simulink model "Comp_FDC_main"  (R2021b)
settings: Solver=FixedStepDiscrete  StartTime=0.0  StopTime=10.0  RelTol=1e-3  EnableMultiTasking=on
settings Model: DataDictionary=APPTypes.sldd  Creator=FVT22063  LastModifiedBy=FVT22063
settings SolverCC: AutoInsertRateTranBlk=on
settings DataIOCC: SaveFormat=StructureWithTime
settings OptimizationCC: DefaultParameterBehavior=Inlined  EnhancedBackFolding=on  PassReuseOutputArgsAs=Individual arguments  ZeroExternalMemoryAtStartup=off  ZeroInternalMemoryAtStartup=off  OptimizeBlockOrder=speed  DifferentSizesBufferReuse=on  OptimizationCustomize=off  EfficientTunableParamExpr=on
settings DebuggingCC: ParameterTunabilityLossMsg=error
settings ModelReferenceCC: ModelReferenceNumInstancesAllowed=Single
settings SFSimCC: MATLABDynamicMemAlloc=off
settings RTWCC: Description=AUTOSAR  SystemTargetFile=autosar.tlc  GenCodeOnly=on  TemplateMakefile=ert_default_tmf
settings CodeAppCC: ForceParamTrailComments=on  IgnoreCustomStorageClasses=off  OperatorAnnotations=on  SimulinkDataObjDesc=on  SFDataObjDesc=on  InsertBlockDesc=on
settings STFCustomTargetCC: TargetLangStandard=C99 (ISO)  MultiwordLength=256  ParMdlRefBuildCompliant=on  CompOptLevelCompliant=on  IncludeMdlTerminateFcn=off  CombineOutputUpdateFcns=on  SuppressErrorStatus=on  ERTCustomFileBanners=on  SupportNonFinite=off  SupportComplex=off  SupportContinuousTime=off  SupportNonInlinedSFcns=off  RemoveResetFunc=on  MATLABClassNameForMDSCustomization=Simulink.SoftwareTarget.ERTCustomization  AutosarCompliant=on  GRTInterface=off  UseToolchainInfoCompliant=on  LookupTableObjectStructAxisOrder=2,1,3,4,...  LUTObjectStructOrderEvenSpacing=Size,Table,Breakpoints  SystemTargetFile=autosar.tlc
settings ERTTargetCC: TargetLangStandard=C99 (ISO)  ConcurrentExecutionCompliant=off  IncludeMdlTerminateFcn=off  SuppressErrorStatus=on  SupportNonFinite=off  SupportComplex=off  ModelStepFunctionPrototypeControlCompliant=off  CPPClassGenCompliant=off  AutosarCompliant=on  LookupTableObjectStructAxisOrder=2,1,3,4,...  LUTObjectStructOrderEvenSpacing=Size,Table,Breakpoints  InlinedParameterPlacement=NonHierarchical  ERTCustomFileTemplate=example_file_process.tlc

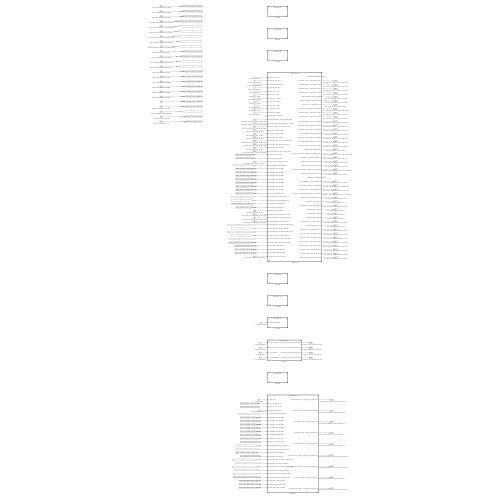
[thumbnail: Simulink's stored preview of the top-level diagram]
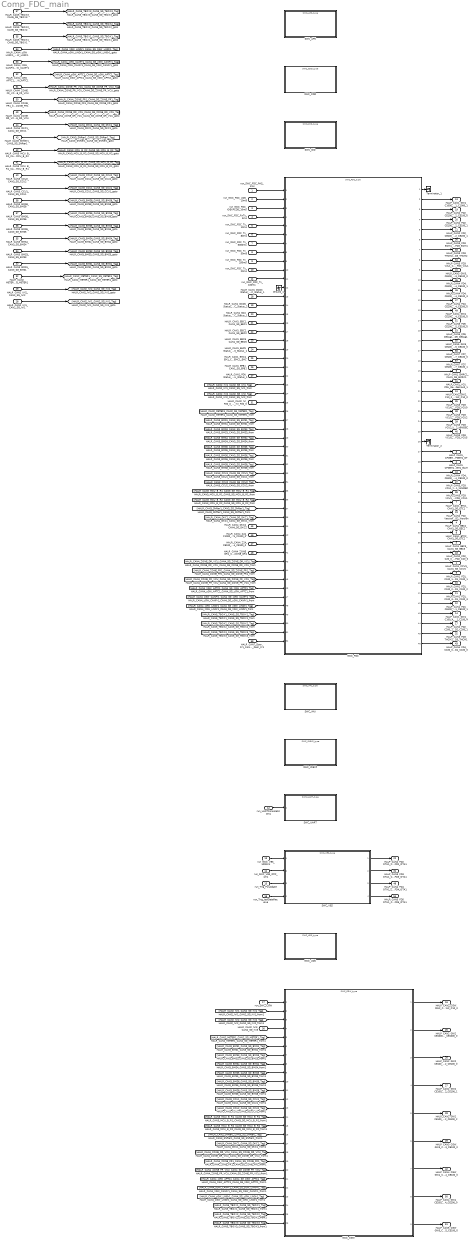
== system Comp_FDC_main ==
  run_SWC_FDC_PAS_1ms : Inport  SampleTime=0.001  OutputFunctionCall=on
  run_SWC_FDC_UDS_10ms : Inport  Port=2  SampleTime=0.01  OutputFunctionCall=on
  run_SWC_FDC_IOEXPCDD_10ms : Inport  Port=3  SampleTime=0.01  OutputFunctionCall=on
  run_SWC_FDC_RxTx_5ms : Inport  Port=4  SampleTime=0.005  OutputFunctionCall=on
  run_SWC_FDC_Tx_10ms : Inport  Port=5  SampleTime=0.01  OutputFunctionCall=on
  run_SWC_FDC_Tx_80ms : Inport  Port=6  SampleTime=0.08  OutputFunctionCall=on
  run_SWC_FDC_Tx_5000ms : Inport  Port=7  SampleTime=5  OutputFunctionCall=on
  run_SWC_FDC_Tx_50ms : Inport  Port=8  SampleTime=0.05  OutputFunctionCall=on
  run_SWC_FDC_Tx_250ms : Inport  Port=9  SampleTime=0.25  OutputFunctionCall=on
  run_SWC_FDC_Tx_20ms : Inport  Port=10  SampleTime=0.02  OutputFunctionCall=on
  run_SWC_FDC_Tx_100ms : Inport  Port=11  SampleTime=0.1  OutputFunctionCall=on
  run_UARTConsole100ms : Inport  Port=12  SampleTime=0.1  OutputFunctionCall=on
  run_SWC_VES_1000ms : Inport  Port=13  SampleTime=1  OutputFunctionCall=on
  run_SWC_VES_IPCF_1ms : Inport  Port=14  SampleTime=0.001  OutputFunctionCall=on
  run_Trig_FwUpdate : Inport  Port=15  OutputFunctionCall=on
  run_Trig_IpcfDataReceive : Inport  Port=16  OutputFunctionCall=on
  run_SWC_CGW : Inport  Port=17  OutputFunctionCall=on
  HALR_CAN1_DCDC_Status_1_CAN1_SG_DCDC_Status_1 : Inport  Port=18  OutDataTypeStr=Bus: DT_CAN1_SG_DCDC_Status_1  PortDimensions=1  BusOutputAsStruct=on
  HALR_CAN1_DCDC_Status_2_CAN1_SG_DCDC_Status_2 : Inport  Port=19  OutDataTypeStr=Bus: DT_CAN1_SG_DCDC_Status_2  PortDimensions=1  BusOutputAsStruct=on
  HALR_CAN1_EAC_Status_1_CAN1_SG_EAC_Status_1 : Inport  Port=20  OutDataTypeStr=Bus: DT_CAN1_SG_EAC_Status_1  PortDimensions=1  BusOutputAsStruct=on
  HALR_CAN1_EBC1_CAN1_SG_EBC1 : Inport  Port=21  OutDataTypeStr=Bus: DT_CAN1_SG_EBC1  PortDimensions=1  BusOutputAsStruct=on
  HALR_CAN1_EBC2_CAN1_SG_EBC2 : Inport  Port=22  OutDataTypeStr=Bus: DT_CAN1_SG_EBC2  PortDimensions=1  BusOutputAsStruct=on
  HALR_CAN1_EBC5_CAN1_SG_EBC5 : Inport  Port=23  OutDataTypeStr=Bus: DT_CAN1_SG_EBC5  PortDimensions=1  BusOutputAsStruct=on
  HALR_CAN1_EHPS_Status_1_CAN1_SG_EHPS_Status_1 : Inport  Port=24  OutDataTypeStr=Bus: DT_CAN1_SG_EHPS_Status_1  PortDimensions=1  BusOutputAsStruct=on
  HALR_CAN1_EMC1_EM1_CAN1_SG_EMC1_EM1 : Inport  Port=25  OutDataTypeStr=Bus: DT_CAN1_SG_EMC1_EM1  PortDimensions=1  BusOutputAsStruct=on
  HALR_CAN1_EPB1_CAN1_SG_EPB1 : Inport  Port=26  OutDataTypeStr=Bus: DT_CAN1_SG_EPB1  PortDimensions=1  BusOutputAsStruct=on
  HALR_CAN1_PDU_Status_1_CAN1_SG_PDU_Status_1 : Inport  Port=27  OutDataTypeStr=Bus: DT_CAN1_SG_PDU_Status_1  PortDimensions=1  BusOutputAsStruct=on
  HALR_CAN2_IVI1_CAN2_SG_IVI1 : Inport  Port=28  OutDataTypeStr=Bus: DT_CAN2_SG_IVI1  PortDimensions=1  BusOutputAsStruct=on
  HALR_CAN2_IVI2_CAN2_SG_IVI2 : Inport  Port=29  OutDataTypeStr=Bus: DT_CAN2_SG_IVI2  PortDimensions=1  BusOutputAsStruct=on
  HALR_CAN2_IVI3_CAN2_SG_IVI3 : Inport  Port=30  OutDataTypeStr=Bus: DT_CAN2_SG_IVI3  PortDimensions=1  BusOutputAsStruct=on
  HALR_CAN2_IVI_P20_0_CAN2_SG_IVI_P20_0 : Inport  Port=31  OutDataTypeStr=Bus: DT_CAN2_SG_IVI_P20_0  PortDimensions=1  BusOutputAsStruct=on
  HALR_CAN2_METER1_CAN2_SG_METER1 : Inport  Port=32  OutDataTypeStr=Bus: DT_CAN2_SG_METER1  PortDimensions=1  BusOutputAsStruct=on
  HALR_CAN3_BMS1_CAN3_SG_BMS1 : Inport  Port=33  OutDataTypeStr=Bus: DT_CAN3_SG_BMS1  PortDimensions=1  BusOutputAsStruct=on
  HALR_CAN3_BMS3_CAN3_SG_BMS3 : Inport  Port=34  OutDataTypeStr=Bus: DT_CAN3_SG_BMS3  PortDimensions=1  BusOutputAsStruct=on
  HALR_CAN3_BMS4_CAN3_SG_BMS4 : Inport  Port=35  OutDataTypeStr=Bus: DT_CAN3_SG_BMS4  PortDimensions=1  BusOutputAsStruct=on
  HALR_CAN3_BMS5_CAN3_SG_BMS5 : Inport  Port=36  OutDataTypeStr=Bus: DT_CAN3_SG_BMS5  PortDimensions=1  BusOutputAsStruct=on
  HALR_CAN3_BMS6_CAN3_SG_BMS6 : Inport  Port=37  OutDataTypeStr=Bus: DT_CAN3_SG_BMS6  PortDimensions=1  BusOutputAsStruct=on
  HALR_CAN3_BMS8_CAN3_SG_BMS8 : Inport  Port=38  OutDataTypeStr=Bus: DT_CAN3_SG_BMS8  PortDimensions=1  BusOutputAsStruct=on
  HALR_CAN3_CCU1_CAN3_SG_CCU1 : Inport  Port=39  OutDataTypeStr=Bus: DT_CAN3_SG_CCU1  PortDimensions=1  BusOutputAsStruct=on
  HALR_CAN3_CCU2_CAN3_SG_CCU2 : Inport  Port=40  OutDataTypeStr=Bus: DT_CAN3_SG_CCU2  PortDimensions=1  BusOutputAsStruct=on
  HALR_CAN3_MCU_B_R1_CAN3_SG_MCU_B_R1 : Inport  Port=41  OutDataTypeStr=Bus: DT_CAN3_SG_MCU_B_R1  PortDimensions=1  BusOutputAsStruct=on
  HALR_CAN3_MCU_B_R2_CAN3_SG_MCU_B_R2 : Inport  Port=42  OutDataTypeStr=Bus: DT_CAN3_SG_MCU_B_R2  PortDimensions=1  BusOutputAsStruct=on
  HALR_CAN3_Shifter1_CAN3_SG_Shifter1 : Inport  Port=43  OutDataTypeStr=Bus: DT_CAN3_SG_Shifter1  PortDimensions=1  BusOutputAsStruct=on
  HALR_CAN4_DKC1_CAN4_SG_DKC1 : Inport  Port=44  OutDataTypeStr=Bus: DT_CAN4_SG_DKC1  PortDimensions=1  BusOutputAsStruct=on
  HALR_CAN4_DKC2_CAN4_SG_DKC2 : Inport  Port=45  OutDataTypeStr=Bus: DT_CAN4_SG_DKC2  PortDimensions=1  BusOutputAsStruct=on
  HALR_CAN4_Z24_C1000_0_CAN4_SG_Z24_C1000_0 : Inport  Port=46  OutDataTypeStr=Bus: DT_CAN4_SG_Z24_C1000_0  PortDimensions=1  BusOutputAsStruct=on
  HALR_CAN4_Z24_CE100_0_CAN4_SG_Z24_CE100_0 : Inport  Port=47  OutDataTypeStr=Bus: DT_CAN4_SG_Z24_CE100_0  PortDimensions=1  BusOutputAsStruct=on
  HALR_CAN4_ZONE_DR1_CAN4_SG_ZONE_DR1 : Inport  Port=48  OutDataTypeStr=Bus: DT_CAN4_SG_ZONE_DR1  PortDimensions=1  BusOutputAsStruct=on
  HALR_CAN4_ZONE_DR_VCU_CAN4_SG_ZONE_DR_VCU : Inport  Port=49  OutDataTypeStr=Bus: DT_CAN4_SG_ZONE_DR_VCU  PortDimensions=1  BusOutputAsStruct=on
  HALR_CAN4_ZONE_FR1_CAN4_SG_ZONE_FR1 : Inport  Port=50  OutDataTypeStr=Bus: DT_CAN4_SG_ZONE_FR1  PortDimensions=1  BusOutputAsStruct=on
  HALR_CAN4_ZONE_FR_VCU_CAN4_SG_ZONE_FR_VCU : Inport  Port=51  OutDataTypeStr=Bus: DT_CAN4_SG_ZONE_FR_VCU  PortDimensions=1  BusOutputAsStruct=on
  HALR_CAN4_zGW_APTC1_CAN4_SG_zGW_APTC1 : Inport  Port=52  OutDataTypeStr=Bus: DT_CAN4_SG_zGW_APTC1  PortDimensions=1  BusOutputAsStruct=on
  HALR_CAN4_zGW_CANFr1_CAN4_SG_zGW_CANFr1 : Inport  Port=53  OutDataTypeStr=Bus: DT_CAN4_SG_zGW_CANFr1  PortDimensions=1  BusOutputAsStruct=on
  HALR_CAN4_zGW_LINDr1_CAN4_SG_zGW_LINDr1 : Inport  Port=54  OutDataTypeStr=Bus: DT_CAN4_SG_zGW_LINDr1  PortDimensions=1  BusOutputAsStruct=on
  HALR_CAN5_TBOX1_CAN5_SG_TBOX1 : Inport  Port=55  OutDataTypeStr=Bus: DT_CAN5_SG_TBOX1  PortDimensions=1  BusOutputAsStruct=on
  HALR_CAN5_TBOX2_CAN5_SG_TBOX2 : Inport  Port=56  OutDataTypeStr=Bus: DT_CAN5_SG_TBOX2  PortDimensions=1  BusOutputAsStruct=on
  HALR_CAN5_TBOX3_CAN5_SG_TBOX3 : Inport  Port=57  OutDataTypeStr=Bus: DT_CAN5_SG_TBOX3  PortDimensions=1  BusOutputAsStruct=on
  HALR_CAN7_Door_Fr1_CAN7_SG_Door_Fr1 : Inport  Port=58  OutDataTypeStr=Bus: DT_CAN7_SG_Door_Fr1  PortDimensions=1  BusOutputAsStruct=on
  Ground_1 : Ground
  SWC_APS : ModelReference  ModelNameDialog=SWC_APS_type  SimulationMode=Normal  ScheduleRates=on  ModelReferenceVersion=1.1
  SWC_CDD : ModelReference  ModelNameDialog=SWC_CDD_type  SimulationMode=Normal  ScheduleRates=on  ModelReferenceVersion=1.1
  SWC_CGW : ModelReference  ModelNameDialog=SWC_CGW_type  SimulationMode=Normal  ScheduleRates=on  ModelReferenceVersion=1.1
  SWC_DID : ModelReference  ModelNameDialog=SWC_DID_type  SimulationMode=Normal  ScheduleRates=on  ModelReferenceVersion=1.1
  SWC_FDC : ModelReference  ModelNameDialog=SWC_FDC_type  SimulationMode=Normal  ScheduleRates=on  ModelReferenceVersion=1.1
  SWC_IMU : ModelReference  ModelNameDialog=SWC_IMU_type  SimulationMode=Normal  ScheduleRates=on  ModelReferenceVersion=1.1
  SWC_IOEXP : ModelReference  ModelNameDialog=SWC_IOEXP_type  SimulationMode=Normal  ScheduleRates=on  ModelReferenceVersion=1.1
  SWC_UART : ModelReference  ModelNameDialog=SWC_UART_type  SimulationMode=Normal  ScheduleRates=on  ModelReferenceVersion=1.1
  SWC_UDS : ModelReference  ModelNameDialog=SWC_UDS_type  SimulationMode=Normal  ScheduleRates=on  ModelReferenceVersion=1.1
  SWC_VES : ModelReference  ModelNameDialog=SWC_VES_type  SimulationMode=Normal  ScheduleRates=on  ModelReferenceVersion=1.1
  Terminator_1 : Terminator
  Terminator_2 : Terminator
  HALP_CAN1_CCVS_CAN1_SG_CCVS : Outport  OutDataTypeStr=Bus: DT_CAN1_SG_CCVS  PortDimensions=1  BusOutputAsStruct=on
  HALP_CAN1_CFGEM1_BAM_CAN1_SG_CFGEM1_BAM : Outport  Port=2  OutDataTypeStr=Bus: DT_CAN1_SG_CFGEM1_BAM  PortDimensions=1  BusOutputAsStruct=on
  HALP_CAN1_CFGEM1_DT_CAN1_SG_CFGEM1_DT : Outport  Port=3  OutDataTypeStr=Bus: DT_CAN1_SG_CFGEM1_DT  PortDimensions=1  BusOutputAsStruct=on
  HALP_CAN1_EEC2_CAN1_SG_EEC2 : Outport  Port=4  OutDataTypeStr=Bus: DT_CAN1_SG_EEC2  PortDimensions=1  BusOutputAsStruct=on
  HALP_CAN1_EEC3_CAN1_SG_EEC3 : Outport  Port=5  OutDataTypeStr=Bus: DT_CAN1_SG_EEC3  PortDimensions=1  BusOutputAsStruct=on
  HALP_CAN1_EMRC1_CAN1_SG_EMRC1 : Outport  Port=6  OutDataTypeStr=Bus: DT_CAN1_SG_EMRC1  PortDimensions=1  BusOutputAsStruct=on
  HALP_CAN1_ETC1_CAN1_SG_ETC1 : Outport  Port=7  OutDataTypeStr=Bus: DT_CAN1_SG_ETC1  PortDimensions=1  BusOutputAsStruct=on
  HALP_CAN1_ETC2_CAN1_SG_ETC2 : Outport  Port=8  OutDataTypeStr=Bus: DT_CAN1_SG_ETC2  PortDimensions=1  BusOutputAsStruct=on
  HALP_CAN1_FD1_C100_1_CAN1_SG_FD1_C100_1 : Outport  Port=9  OutDataTypeStr=Bus: DT_CAN1_SG_FD1_C100_1  PortDimensions=1  BusOutputAsStruct=on
  HALP_CAN1_FD1_C100_2_CAN1_SG_FD1_C100_2 : Outport  Port=10  OutDataTypeStr=Bus: DT_CAN1_SG_FD1_C100_2  PortDimensions=1  BusOutputAsStruct=on
  HALP_CAN1_FD1_C100_3_CAN1_SG_FD1_C100_3 : Outport  Port=11  OutDataTypeStr=Bus: DT_CAN1_SG_FD1_C100_3  PortDimensions=1  BusOutputAsStruct=on
  HALP_CAN1_FD1_CE100_1_CAN1_SG_FD1_CE100_1 : Outport  Port=12  OutDataTypeStr=Bus: DT_CAN1_SG_FD1_CE100_1  PortDimensions=1  BusOutputAsStruct=on
  HALP_CAN1_GW1_C1000_1_CAN1_SG_GW1_C1000_1 : Outport  Port=13  OutDataTypeStr=Bus: DT_CAN1_SG_GW1_C1000_1  PortDimensions=1  BusOutputAsStruct=on
  HALP_CAN1_GW1_C100_4_CAN1_SG_GW1_C100_4 : Outport  Port=14  OutDataTypeStr=Bus: DT_CAN1_SG_GW1_C100_4  PortDimensions=1  BusOutputAsStruct=on
  HALP_CAN1_VCU_PDU_Demand_1_CAN1_SG_VCU_PDU_Demand_1 : Outport  Port=15  OutDataTypeStr=Bus: DT_CAN1_SG_VCU_PDU_Demand_1  PortDimensions=1  BusOutputAsStruct=on
  HALP_CAN2_CGW_GW2_C10_0_CAN2_SG_CGW_GW2_C10_0 : Outport  Port=16  OutDataTypeStr=Bus: DT_CAN2_SG_CGW_GW2_C10_0  PortDimensions=1  BusOutputAsStruct=on
  HALP_CAN2_FD2_C200_1_CAN2_SG_FD2_C200_1 : Outport  Port=17  OutDataTypeStr=Bus: DT_CAN2_SG_FD2_C200_1  PortDimensions=1  BusOutputAsStruct=on
  HALP_CAN2_FD2_C20_0_CAN2_SG_FD2_C20_0 : Outport  Port=18  OutDataTypeStr=Bus: DT_CAN2_SG_FD2_C20_0  PortDimensions=1  BusOutputAsStruct=on
  HALP_CAN2_FD2_CE100_0_CAN2_SG_FD2_CE100_0 : Outport  Port=19  OutDataTypeStr=Bus: DT_CAN2_SG_FD2_CE100_0  PortDimensions=1  BusOutputAsStruct=on
  HALP_CAN2_FD2_CE100_1_CAN2_SG_FD2_CE100_1 : Outport  Port=20  OutDataTypeStr=Bus: DT_CAN2_SG_FD2_CE100_1  PortDimensions=1  BusOutputAsStruct=on
  HALP_CAN2_FD2_CE200_1_CAN2_SG_FD2_CE200_1 : Outport  Port=21  OutDataTypeStr=Bus: DT_CAN2_SG_FD2_CE200_1  PortDimensions=1  BusOutputAsStruct=on
  HALP_CAN2_FD2_OTA1_CAN2_SG_FD2_OTA1 : Outport  Port=22  OutDataTypeStr=Bus: DT_CAN2_SG_FD2_OTA1  PortDimensions=1  BusOutputAsStruct=on
  HALP_CAN2_FD2_Version_CAN2_SG_FD2_Version : Outport  Port=23  OutDataTypeStr=Bus: DT_CAN2_SG_FD2_Version  PortDimensions=1  BusOutputAsStruct=on
  HALP_CAN2_GW2_C10_0_CAN2_SG_GW2_C10_0 : Outport  Port=24  OutDataTypeStr=Bus: DT_CAN2_SG_GW2_C10_0  PortDimensions=1  BusOutputAsStruct=on
  HALP_CAN2_GW2_CE1000_0_CAN2_SG_GW2_CE1000_0 : Outport  Port=25  OutDataTypeStr=Bus: DT_CAN2_SG_GW2_CE1000_0  PortDimensions=1  BusOutputAsStruct=on
  HALP_CAN2_GW2_CE100_0_CAN2_SG_GW2_CE100_0 : Outport  Port=26  OutDataTypeStr=Bus: DT_CAN2_SG_GW2_CE100_0  PortDimensions=1  BusOutputAsStruct=on
  HALP_CAN2_GW2_CE100_1_CAN2_SG_GW2_CE100_1 : Outport  Port=27  OutDataTypeStr=Bus: DT_CAN2_SG_GW2_CE100_1  PortDimensions=1  BusOutputAsStruct=on
  HALP_CAN2_GW2_CE100_2_CAN2_SG_GW2_CE100_2 : Outport  Port=28  OutDataTypeStr=Bus: DT_CAN2_SG_GW2_CE100_2  PortDimensions=1  BusOutputAsStruct=on
  HALP_CAN3_CGW_GW3_CE100_0_CAN3_SG_CGW_GW3_CE100_0 : Outport  Port=29  OutDataTypeStr=Bus: DT_CAN3_SG_CGW_GW3_CE100_0  PortDimensions=1  BusOutputAsStruct=on
  HALP_CAN3_FD3_BCM1_CAN3_SG_FD3_BCM1 : Outport  Port=30  OutDataTypeStr=Bus: DT_CAN3_SG_FD3_BCM1  PortDimensions=1  BusOutputAsStruct=on
  HALP_CAN3_FD3_OTA1_CAN3_SG_FD3_OTA1 : Outport  Port=31  OutDataTypeStr=Bus: DT_CAN3_SG_FD3_OTA1  PortDimensions=1  BusOutputAsStruct=on
  HALP_CAN3_FD3_THCM1_CAN3_SG_FD3_THCM1 : Outport  Port=32  OutDataTypeStr=Bus: DT_CAN3_SG_FD3_THCM1  PortDimensions=1  BusOutputAsStruct=on
  HALP_CAN3_FD3_THCM2_CAN3_SG_FD3_THCM2 : Outport  Port=33  OutDataTypeStr=Bus: DT_CAN3_SG_FD3_THCM2  PortDimensions=1  BusOutputAsStruct=on
  HALP_CAN3_FD3_V2L1_CAN3_SG_FD3_V2L1 : Outport  Port=34  OutDataTypeStr=Bus: DT_CAN3_SG_FD3_V2L1  PortDimensions=1  BusOutputAsStruct=on
  HALP_CAN3_FD3_VCU0_CAN3_SG_FD3_VCU0 : Outport  Port=35  OutDataTypeStr=Bus: DT_CAN3_SG_FD3_VCU0  PortDimensions=1  BusOutputAsStruct=on
  HALP_CAN3_FD3_VCU1_CAN3_SG_FD3_VCU1 : Outport  Port=36  OutDataTypeStr=Bus: DT_CAN3_SG_FD3_VCU1  PortDimensions=1  BusOutputAsStruct=on
  HALP_CAN3_FD3_VCU1_toNIDEC_CAN3_SG_FD3_VCU1_toNIDEC : Outport  Port=37  OutDataTypeStr=Bus: DT_CAN3_SG_FD3_VCU1_toNIDEC  PortDimensions=1  BusOutputAsStruct=on
  HALP_CAN3_FD3_VCU2_CAN3_SG_FD3_VCU2 : Outport  Port=38  OutDataTypeStr=Bus: DT_CAN3_SG_FD3_VCU2  PortDimensions=1  BusOutputAsStruct=on
  HALP_CAN3_FD3_VCU2_toNIDEC_CAN3_SG_FD3_VCU2_toNIDEC : Outport  Port=39  OutDataTypeStr=Bus: DT_CAN3_SG_FD3_VCU2_toNIDEC  PortDimensions=1  BusOutputAsStruct=on
  HALP_CAN3_FD3_VCU5_CAN3_SG_FD3_VCU5 : Outport  Port=40  OutDataTypeStr=Bus: DT_CAN3_SG_FD3_VCU5  PortDimensions=1  BusOutputAsStruct=on
  HALP_CAN3_GW3_CE100_0_CAN3_SG_GW3_CE100_0 : Outport  Port=41  OutDataTypeStr=Bus: DT_CAN3_SG_GW3_CE100_0  PortDimensions=1  BusOutputAsStruct=on
  HALP_CAN4_CGW_GW4_CE100_0_CAN4_SG_CGW_GW4_CE100_0 : Outport  Port=42  OutDataTypeStr=Bus: DT_CAN4_SG_CGW_GW4_CE100_0  PortDimensions=1  BusOutputAsStruct=on
  HALP_CAN4_FD4_C100_0_CAN4_SG_FD4_C100_0 : Outport  Port=43  OutDataTypeStr=Bus: DT_CAN4_SG_FD4_C100_0  PortDimensions=1  BusOutputAsStruct=on
  HALP_CAN4_FD4_CE100_0_CAN4_SG_FD4_CE100_0 : Outport  Port=44  OutDataTypeStr=Bus: DT_CAN4_SG_FD4_CE100_0  PortDimensions=1  BusOutputAsStruct=on
  HALP_CAN4_FD4_CE100_1_CAN4_SG_FD4_CE100_1 : Outport  Port=45  OutDataTypeStr=Bus: DT_CAN4_SG_FD4_CE100_1  PortDimensions=1  BusOutputAsStruct=on
  HALP_CAN4_FD4_CE100_3_CAN4_SG_FD4_CE100_3 : Outport  Port=46  OutDataTypeStr=Bus: DT_CAN4_SG_FD4_CE100_3  PortDimensions=1  BusOutputAsStruct=on
  HALP_CAN4_FD4_CE200_0_CAN4_SG_FD4_CE200_0 : Outport  Port=47  OutDataTypeStr=Bus: DT_CAN4_SG_FD4_CE200_0  PortDimensions=1  BusOutputAsStruct=on
  HALP_CAN4_FD4_OTA1_CAN4_SG_FD4_OTA1 : Outport  Port=48  OutDataTypeStr=Bus: DT_CAN4_SG_FD4_OTA1  PortDimensions=1  BusOutputAsStruct=on
  HALP_CAN4_GW4_CE100_0_CAN4_SG_GW4_CE100_0 : Outport  Port=49  OutDataTypeStr=Bus: DT_CAN4_SG_GW4_CE100_0  PortDimensions=1  BusOutputAsStruct=on
  HALP_CAN4_GW4_CE200_0_CAN4_SG_GW4_CE200_0 : Outport  Port=50  OutDataTypeStr=Bus: DT_CAN4_SG_GW4_CE200_0  PortDimensions=1  BusOutputAsStruct=on
  HALP_CAN5_CGW_GW5_CE100_0_CAN5_SG_CGW_GW5_CE100_0 : Outport  Port=51  OutDataTypeStr=Bus: DT_CAN5_SG_CGW_GW5_CE100_0  PortDimensions=1  BusOutputAsStruct=on
  HALP_CAN5_FD5_CE100_0_CAN5_SG_FD5_CE100_0 : Outport  Port=52  OutDataTypeStr=Bus: DT_CAN5_SG_FD5_CE100_0  PortDimensions=1  BusOutputAsStruct=on
  HALP_CAN5_FD5_Debug1_CAN5_SG_FD5_Debug1 : Outport  Port=53  OutDataTypeStr=Bus: DT_CAN5_SG_FD5_Debug1  PortDimensions=1  BusOutputAsStruct=on
  HALP_CAN5_FD5_OTA1_CAN5_SG_FD5_OTA1 : Outport  Port=54  OutDataTypeStr=Bus: DT_CAN5_SG_FD5_OTA1  PortDimensions=1  BusOutputAsStruct=on
  HALP_CAN5_GW5_CE100_0_CAN5_SG_GW5_CE100_0 : Outport  Port=55  OutDataTypeStr=Bus: DT_CAN5_SG_GW5_CE100_0  PortDimensions=1  BusOutputAsStruct=on
  HALP_CAN7_FD7_CE100_0_CAN7_SG_FD7_CE100_0 : Outport  Port=56  OutDataTypeStr=Bus: DT_CAN7_SG_FD7_CE100_0  PortDimensions=1  BusOutputAsStruct=on
  HALP_CAN7_FD7_CE100_1_CAN7_SG_FD7_CE100_1 : Outport  Port=57  OutDataTypeStr=Bus: DT_CAN7_SG_FD7_CE100_1  PortDimensions=1  BusOutputAsStruct=on
  wires:
  run_SWC_FDC_PAS_1ms/1 -> SWC_FDC/1
  run_SWC_FDC_UDS_10ms/1 -> SWC_FDC/2
  run_SWC_FDC_IOEXPCDD_10ms/1 -> SWC_FDC/3
  run_SWC_FDC_RxTx_5ms/1 -> SWC_FDC/4
  run_SWC_FDC_Tx_10ms/1 -> SWC_FDC/5
  run_SWC_FDC_Tx_80ms/1 -> SWC_FDC/6
  run_SWC_FDC_Tx_5000ms/1 -> SWC_FDC/7
  run_SWC_FDC_Tx_50ms/1 -> SWC_FDC/8
  run_SWC_FDC_Tx_250ms/1 -> SWC_FDC/9
  run_SWC_FDC_Tx_20ms/1 -> SWC_FDC/10
  run_SWC_FDC_Tx_100ms/1 -> SWC_FDC/11
  run_UARTConsole100ms/1 -> SWC_UART/1
  run_SWC_VES_1000ms/1 -> SWC_VES/1
  run_SWC_VES_IPCF_1ms/1 -> SWC_VES/2
  run_Trig_FwUpdate/1 -> SWC_VES/3
  run_Trig_IpcfDataReceive/1 -> SWC_VES/4
  run_SWC_CGW/1 -> SWC_CGW/1
  HALR_CAN1_DCDC_Status_1_CAN1_SG_DCDC_Status_1/1 -> SWC_FDC/13
  HALR_CAN1_DCDC_Status_2_CAN1_SG_DCDC_Status_2/1 -> SWC_FDC/14
  HALR_CAN1_EAC_Status_1_CAN1_SG_EAC_Status_1/1 -> SWC_FDC/15
  HALR_CAN1_EBC1_CAN1_SG_EBC1/1 -> SWC_FDC/16
  HALR_CAN1_EBC2_CAN1_SG_EBC2/1 -> SWC_FDC/17
  HALR_CAN1_EBC5_CAN1_SG_EBC5/1 -> SWC_FDC/18
  HALR_CAN1_EHPS_Status_1_CAN1_SG_EHPS_Status_1/1 -> SWC_FDC/19
  HALR_CAN1_EMC1_EM1_CAN1_SG_EMC1_EM1/1 -> SWC_FDC/20
  HALR_CAN1_EPB1_CAN1_SG_EPB1/1 -> SWC_FDC/21
  HALR_CAN1_PDU_Status_1_CAN1_SG_PDU_Status_1/1 -> SWC_FDC/22
  HALR_CAN2_IVI_P20_0_CAN2_SG_IVI_P20_0/1 -> SWC_FDC/25
  HALR_CAN4_DKC2_CAN4_SG_DKC2/1 -> SWC_FDC/39
  HALR_CAN4_Z24_C1000_0_CAN4_SG_Z24_C1000_0/1 -> SWC_FDC/40
  HALR_CAN4_Z24_CE100_0_CAN4_SG_Z24_CE100_0/1 -> SWC_FDC/41
  HALR_CAN4_ZONE_DR1_CAN4_SG_ZONE_DR1/1 -> SWC_FDC/42
  HALR_CAN7_Door_Fr1_CAN7_SG_Door_Fr1/1 -> SWC_FDC/52
  HALR_CAN2_IVI3_CAN2_SG_IVI3/1 -> SWC_CGW/4
  SWC_FDC/38 -> HALP_CAN1_CCVS_CAN1_SG_CCVS/1
  SWC_FDC/28 -> HALP_CAN1_CFGEM1_BAM_CAN1_SG_CFGEM1_BAM/1
  SWC_FDC/27 -> HALP_CAN1_CFGEM1_DT_CAN1_SG_CFGEM1_DT/1
  SWC_FDC/34 -> HALP_CAN1_EEC2_CAN1_SG_EEC2/1
  SWC_FDC/36 -> HALP_CAN1_EEC3_CAN1_SG_EEC3/1
  SWC_FDC/19 -> HALP_CAN1_EMRC1_CAN1_SG_EMRC1/1
  SWC_FDC/32 -> HALP_CAN1_ETC1_CAN1_SG_ETC1/1
  SWC_FDC/35 -> HALP_CAN1_ETC2_CAN1_SG_ETC2/1
  SWC_FDC/39 -> HALP_CAN1_FD1_C100_1_CAN1_SG_FD1_C100_1/1
  SWC_FDC/40 -> HALP_CAN1_FD1_C100_2_CAN1_SG_FD1_C100_2/1
  SWC_FDC/41 -> HALP_CAN1_FD1_C100_3_CAN1_SG_FD1_C100_3/1
  SWC_FDC/42 -> HALP_CAN1_FD1_CE100_1_CAN1_SG_FD1_CE100_1/1
  SWC_FDC/2 -> HALP_CAN1_GW1_C1000_1_CAN1_SG_GW1_C1000_1/1
  SWC_FDC/43 -> HALP_CAN1_GW1_C100_4_CAN1_SG_GW1_C100_4/1
  SWC_FDC/20 -> HALP_CAN1_VCU_PDU_Demand_1_CAN1_SG_VCU_PDU_Demand_1/1
  SWC_FDC/44 -> HALP_CAN2_FD2_C200_1_CAN2_SG_FD2_C200_1/1
  SWC_FDC/37 -> HALP_CAN2_FD2_C20_0_CAN2_SG_FD2_C20_0/1
  SWC_FDC/3 -> HALP_CAN2_FD2_CE100_0_CAN2_SG_FD2_CE100_0/1
  SWC_FDC/4 -> HALP_CAN2_FD2_CE100_1_CAN2_SG_FD2_CE100_1/1
  SWC_FDC/5 -> HALP_CAN2_FD2_CE200_1_CAN2_SG_FD2_CE200_1/1
  SWC_VES/1 -> HALP_CAN2_FD2_OTA1_CAN2_SG_FD2_OTA1/1
  SWC_FDC/33 -> HALP_CAN2_FD2_Version_CAN2_SG_FD2_Version/1
  SWC_FDC/21 -> HALP_CAN2_GW2_C10_0_CAN2_SG_GW2_C10_0/1
  SWC_FDC/6 -> HALP_CAN3_FD3_BCM1_CAN3_SG_FD3_BCM1/1
  SWC_VES/2 -> HALP_CAN3_FD3_OTA1_CAN3_SG_FD3_OTA1/1
  SWC_FDC/45 -> HALP_CAN3_FD3_THCM1_CAN3_SG_FD3_THCM1/1
  SWC_FDC/7 -> HALP_CAN3_FD3_THCM2_CAN3_SG_FD3_THCM2/1
  SWC_FDC/8 -> HALP_CAN3_FD3_V2L1_CAN3_SG_FD3_V2L1/1
  SWC_FDC/22 -> HALP_CAN3_FD3_VCU0_CAN3_SG_FD3_VCU0/1
  SWC_FDC/31 -> HALP_CAN3_FD3_VCU1_CAN3_SG_FD3_VCU1/1
  SWC_FDC/30 -> HALP_CAN3_FD3_VCU1_toNIDEC_CAN3_SG_FD3_VCU1_toNIDEC/1
  SWC_FDC/23 -> HALP_CAN3_FD3_VCU2_CAN3_SG_FD3_VCU2/1
  SWC_FDC/24 -> HALP_CAN3_FD3_VCU2_toNIDEC_CAN3_SG_FD3_VCU2_toNIDEC/1
  SWC_FDC/25 -> HALP_CAN3_FD3_VCU5_CAN3_SG_FD3_VCU5/1
  SWC_FDC/9 -> HALP_CAN3_GW3_CE100_0_CAN3_SG_GW3_CE100_0/1
  SWC_FDC/46 -> HALP_CAN4_FD4_C100_0_CAN4_SG_FD4_C100_0/1
  SWC_FDC/29 -> HALP_CAN4_FD4_CE100_0_CAN4_SG_FD4_CE100_0/1
  SWC_FDC/10 -> HALP_CAN4_FD4_CE100_1_CAN4_SG_FD4_CE100_1/1
  SWC_FDC/11 -> HALP_CAN4_FD4_CE100_3_CAN4_SG_FD4_CE100_3/1
  SWC_FDC/12 -> HALP_CAN4_FD4_CE200_0_CAN4_SG_FD4_CE200_0/1
  SWC_VES/3 -> HALP_CAN4_FD4_OTA1_CAN4_SG_FD4_OTA1/1
  SWC_FDC/13 -> HALP_CAN4_GW4_CE100_0_CAN4_SG_GW4_CE100_0/1
  SWC_FDC/14 -> HALP_CAN5_FD5_CE100_0_CAN5_SG_FD5_CE100_0/1
  SWC_FDC/15 -> HALP_CAN5_FD5_Debug1_CAN5_SG_FD5_Debug1/1
  SWC_VES/4 -> HALP_CAN5_FD5_OTA1_CAN5_SG_FD5_OTA1/1
  SWC_FDC/16 -> HALP_CAN5_GW5_CE100_0_CAN5_SG_GW5_CE100_0/1
  SWC_FDC/17 -> HALP_CAN7_FD7_CE100_0_CAN7_SG_FD7_CE100_0/1
  SWC_FDC/18 -> HALP_CAN7_FD7_CE100_1_CAN7_SG_FD7_CE100_1/1
  SWC_CGW/1 -> HALP_CAN2_CGW_GW2_C10_0_CAN2_SG_CGW_GW2_C10_0/1
  SWC_CGW/2 -> HALP_CAN2_GW2_CE1000_0_CAN2_SG_GW2_CE1000_0/1
  SWC_CGW/3 -> HALP_CAN2_GW2_CE100_0_CAN2_SG_GW2_CE100_0/1
  SWC_CGW/4 -> HALP_CAN2_GW2_CE100_1_CAN2_SG_GW2_CE100_1/1
  SWC_CGW/5 -> HALP_CAN2_GW2_CE100_2_CAN2_SG_GW2_CE100_2/1
  SWC_CGW/6 -> HALP_CAN3_CGW_GW3_CE100_0_CAN3_SG_CGW_GW3_CE100_0/1
  SWC_CGW/7 -> HALP_CAN4_CGW_GW4_CE100_0_CAN4_SG_CGW_GW4_CE100_0/1
  SWC_CGW/8 -> HALP_CAN4_GW4_CE200_0_CAN4_SG_GW4_CE200_0/1
  SWC_CGW/9 -> HALP_CAN5_CGW_GW5_CE100_0_CAN5_SG_CGW_GW5_CE100_0/1
  HALR_CAN5_TBOX3_CAN5_SG_TBOX3/1 -> [HALR_CAN5_TBOX3_CAN5_SG_TBOX3_Tag]
  [HALR_CAN5_TBOX3_CAN5_SG_TBOX3_Tag] -> SWC_FDC/51
  [HALR_CAN5_TBOX3_CAN5_SG_TBOX3_Tag] -> SWC_CGW/26
  HALR_CAN5_TBOX2_CAN5_SG_TBOX2/1 -> [HALR_CAN5_TBOX2_CAN5_SG_TBOX2_Tag]
  [HALR_CAN5_TBOX2_CAN5_SG_TBOX2_Tag] -> SWC_FDC/50
  [HALR_CAN5_TBOX2_CAN5_SG_TBOX2_Tag] -> SWC_CGW/25
  HALR_CAN5_TBOX1_CAN5_SG_TBOX1/1 -> [HALR_CAN5_TBOX1_CAN5_SG_TBOX1_Tag]
  [HALR_CAN5_TBOX1_CAN5_SG_TBOX1_Tag] -> SWC_FDC/49
  [HALR_CAN5_TBOX1_CAN5_SG_TBOX1_Tag] -> SWC_CGW/24
  HALR_CAN4_zGW_LINDr1_CAN4_SG_zGW_LINDr1/1 -> [HALR_CAN4_zGW_LINDr1_CAN4_SG_zGW_LINDr1_Tag]
  [HALR_CAN4_zGW_LINDr1_CAN4_SG_zGW_LINDr1_Tag] -> SWC_FDC/48
  [HALR_CAN4_zGW_LINDr1_CAN4_SG_zGW_LINDr1_Tag] -> SWC_CGW/23
  HALR_CAN4_zGW_CANFr1_CAN4_SG_zGW_CANFr1/1 -> [HALR_CAN4_zGW_CANFr1_CAN4_SG_zGW_CANFr1_Tag]
  [HALR_CAN4_zGW_CANFr1_CAN4_SG_zGW_CANFr1_Tag] -> SWC_FDC/47
  [HALR_CAN4_zGW_CANFr1_CAN4_SG_zGW_CANFr1_Tag] -> SWC_CGW/22
  HALR_CAN4_zGW_APTC1_CAN4_SG_zGW_APTC1/1 -> [HALR_CAN4_zGW_APTC1_CAN4_SG_zGW_APTC1_Tag]
  [HALR_CAN4_zGW_APTC1_CAN4_SG_zGW_APTC1_Tag] -> SWC_FDC/46
  [HALR_CAN4_zGW_APTC1_CAN4_SG_zGW_APTC1_Tag] -> SWC_CGW/21
  HALR_CAN4_ZONE_FR_VCU_CAN4_SG_ZONE_FR_VCU/1 -> [HALR_CAN4_ZONE_FR_VCU_CAN4_SG_ZONE_FR_VCU_Tag]
  [HALR_CAN4_ZONE_FR_VCU_CAN4_SG_ZONE_FR_VCU_Tag] -> SWC_FDC/45
  [HALR_CAN4_ZONE_FR_VCU_CAN4_SG_ZONE_FR_VCU_Tag] -> SWC_CGW/20
  HALR_CAN4_ZONE_FR1_CAN4_SG_ZONE_FR1/1 -> [HALR_CAN4_ZONE_FR1_CAN4_SG_ZONE_FR1_Tag]
  [HALR_CAN4_ZONE_FR1_CAN4_SG_ZONE_FR1_Tag] -> SWC_FDC/44
  [HALR_CAN4_ZONE_FR1_CAN4_SG_ZONE_FR1_Tag] -> SWC_CGW/19
  HALR_CAN4_ZONE_DR_VCU_CAN4_SG_ZONE_DR_VCU/1 -> [HALR_CAN4_ZONE_DR_VCU_CAN4_SG_ZONE_DR_VCU_Tag]
  [HALR_CAN4_ZONE_DR_VCU_CAN4_SG_ZONE_DR_VCU_Tag] -> SWC_FDC/43
  [HALR_CAN4_ZONE_DR_VCU_CAN4_SG_ZONE_DR_VCU_Tag] -> SWC_CGW/18
  HALR_CAN4_DKC1_CAN4_SG_DKC1/1 -> [HALR_CAN4_DKC1_CAN4_SG_DKC1_Tag]
  [HALR_CAN4_DKC1_CAN4_SG_DKC1_Tag] -> SWC_FDC/38
  [HALR_CAN4_DKC1_CAN4_SG_DKC1_Tag] -> SWC_CGW/17
  HALR_CAN3_Shifter1_CAN3_SG_Shifter1/1 -> [HALR_CAN3_Shifter1_CAN3_SG_Shifter1_Tag]
  [HALR_CAN3_Shifter1_CAN3_SG_Shifter1_Tag] -> SWC_FDC/37
  [HALR_CAN3_Shifter1_CAN3_SG_Shifter1_Tag] -> SWC_CGW/16
  HALR_CAN3_MCU_B_R2_CAN3_SG_MCU_B_R2/1 -> [HALR_CAN3_MCU_B_R2_CAN3_SG_MCU_B_R2_Tag]
  [HALR_CAN3_MCU_B_R2_CAN3_SG_MCU_B_R2_Tag] -> SWC_FDC/36
  [HALR_CAN3_MCU_B_R2_CAN3_SG_MCU_B_R2_Tag] -> SWC_CGW/15
  HALR_CAN3_MCU_B_R1_CAN3_SG_MCU_B_R1/1 -> [HALR_CAN3_MCU_B_R1_CAN3_SG_MCU_B_R1_Tag]
  [HALR_CAN3_MCU_B_R1_CAN3_SG_MCU_B_R1_Tag] -> SWC_FDC/35
  [HALR_CAN3_MCU_B_R1_CAN3_SG_MCU_B_R1_Tag] -> SWC_CGW/14
  HALR_CAN3_CCU2_CAN3_SG_CCU2/1 -> [HALR_CAN3_CCU2_CAN3_SG_CCU2_Tag]
  [HALR_CAN3_CCU2_CAN3_SG_CCU2_Tag] -> SWC_FDC/34
  [HALR_CAN3_CCU2_CAN3_SG_CCU2_Tag] -> SWC_CGW/13
  HALR_CAN3_CCU1_CAN3_SG_CCU1/1 -> [HALR_CAN3_CCU1_CAN3_SG_CCU1_Tag]
  [HALR_CAN3_CCU1_CAN3_SG_CCU1_Tag] -> SWC_FDC/33
  [HALR_CAN3_CCU1_CAN3_SG_CCU1_Tag] -> SWC_CGW/12
  HALR_CAN3_BMS8_CAN3_SG_BMS8/1 -> [HALR_CAN3_BMS8_CAN3_SG_BMS8_Tag]
  [HALR_CAN3_BMS8_CAN3_SG_BMS8_Tag] -> SWC_FDC/32
  [HALR_CAN3_BMS8_CAN3_SG_BMS8_Tag] -> SWC_CGW/11
  HALR_CAN3_BMS6_CAN3_SG_BMS6/1 -> [HALR_CAN3_BMS6_CAN3_SG_BMS6_Tag]
  [HALR_CAN3_BMS6_CAN3_SG_BMS6_Tag] -> SWC_FDC/31
  [HALR_CAN3_BMS6_CAN3_SG_BMS6_Tag] -> SWC_CGW/10
  HALR_CAN3_BMS5_CAN3_SG_BMS5/1 -> [HALR_CAN3_BMS5_CAN3_SG_BMS5_Tag]
  [HALR_CAN3_BMS5_CAN3_SG_BMS5_Tag] -> SWC_FDC/30
  [HALR_CAN3_BMS5_CAN3_SG_BMS5_Tag] -> SWC_CGW/9
  HALR_CAN3_BMS4_CAN3_SG_BMS4/1 -> [HALR_CAN3_BMS4_CAN3_SG_BMS4_Tag]
  [HALR_CAN3_BMS4_CAN3_SG_BMS4_Tag] -> SWC_FDC/29
  [HALR_CAN3_BMS4_CAN3_SG_BMS4_Tag] -> SWC_CGW/8
  HALR_CAN3_BMS3_CAN3_SG_BMS3/1 -> [HALR_CAN3_BMS3_CAN3_SG_BMS3_Tag]
  [HALR_CAN3_BMS3_CAN3_SG_BMS3_Tag] -> SWC_FDC/28
  [HALR_CAN3_BMS3_CAN3_SG_BMS3_Tag] -> SWC_CGW/7
  HALR_CAN3_BMS1_CAN3_SG_BMS1/1 -> [HALR_CAN3_BMS1_CAN3_SG_BMS1_Tag]
  [HALR_CAN3_BMS1_CAN3_SG_BMS1_Tag] -> SWC_FDC/27
  [HALR_CAN3_BMS1_CAN3_SG_BMS1_Tag] -> SWC_CGW/6
  HALR_CAN2_METER1_CAN2_SG_METER1/1 -> [HALR_CAN2_METER1_CAN2_SG_METER1_Tag]
  [HALR_CAN2_METER1_CAN2_SG_METER1_Tag] -> SWC_FDC/26
  [HALR_CAN2_METER1_CAN2_SG_METER1_Tag] -> SWC_CGW/5
  HALR_CAN2_IVI2_CAN2_SG_IVI2/1 -> [HALR_CAN2_IVI2_CAN2_SG_IVI2_Tag]
  [HALR_CAN2_IVI2_CAN2_SG_IVI2_Tag] -> SWC_FDC/24
  [HALR_CAN2_IVI2_CAN2_SG_IVI2_Tag] -> SWC_CGW/3
  HALR_CAN2_IVI1_CAN2_SG_IVI1/1 -> [HALR_CAN2_IVI1_CAN2_SG_IVI1_Tag]
  [HALR_CAN2_IVI1_CAN2_SG_IVI1_Tag] -> SWC_FDC/23
  [HALR_CAN2_IVI1_CAN2_SG_IVI1_Tag] -> SWC_CGW/2
  Ground_1/1 -> SWC_FDC/12
  SWC_FDC/1 -> Terminator_1/1
  SWC_FDC/26 -> Terminator_2/1
